simulink model "model_0"  (R2023b)
settings: Solver=VariableStepAuto  StartTime=0.0  StopTime=50  RelTol=1e-3
values from neighbouring files (symbols this model uses):
  is_zero = false    [init.m]
  k_0 = 1    [init.m]    (also in init8.m = 7)
  k_M_0 = 25    [init.m]    (also in init8.m)
  k_M_1 = 10    [init.m]    (also in init8.m)
settings Model: Creator=lalayants  LastModifiedBy=lalayants

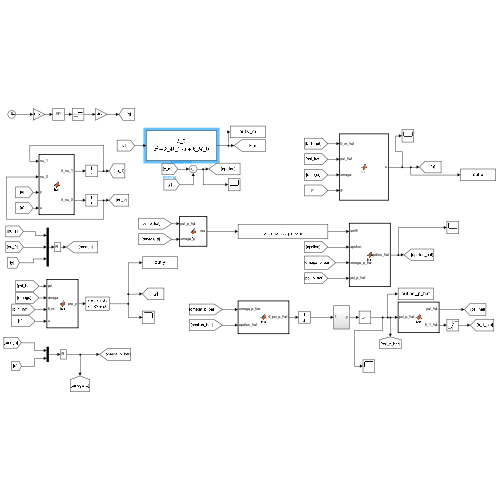
[thumbnail: Simulink's stored preview of the top-level diagram]
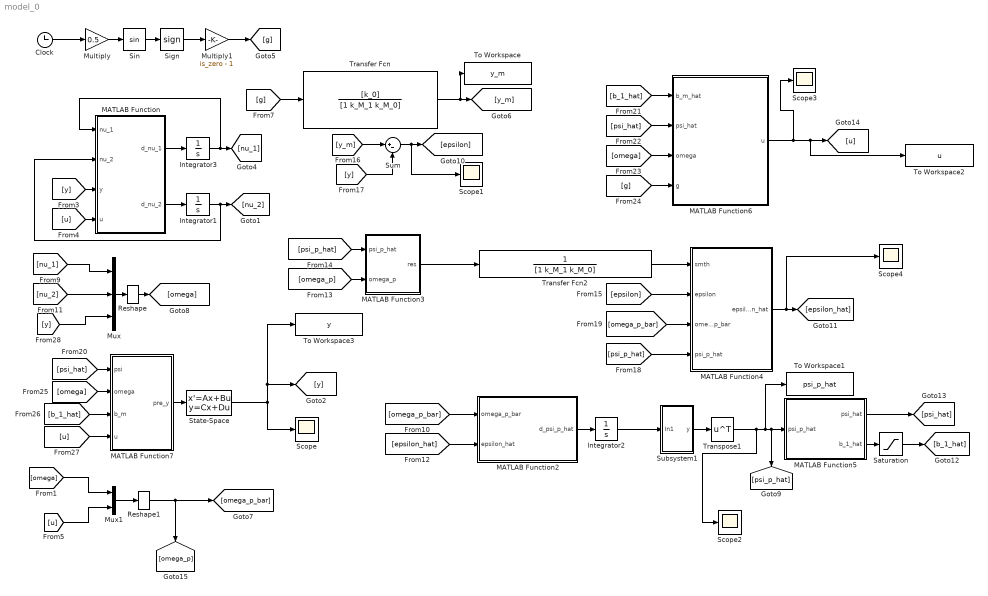
== system model_0 ==
  Clock : Clock
  Integrator1 : Integrator
  Integrator2 : Integrator  InitialCondition=[10; 10; 10; 10]
  Integrator3 : Integrator
  MATLAB Function : MATLAB Function  TreatAsAtomicUnit=on
  MATLAB Function2 : MATLAB Function  TreatAsAtomicUnit=on
  MATLAB Function3 : MATLAB Function  TreatAsAtomicUnit=on
  MATLAB Function4 : MATLAB Function  TreatAsAtomicUnit=on
  MATLAB Function5 : MATLAB Function  TreatAsAtomicUnit=on
  MATLAB Function6 : MATLAB Function  TreatAsAtomicUnit=on
  MATLAB Function7 : MATLAB Function  TreatAsAtomicUnit=on
  Multiply : Gain  Gain=0.5
  Multiply1 : Gain  Gain=is_zero - 1
  Mux : Mux  Inputs=3
  Mux1 : Mux  Inputs=2
  Reshape : Reshape  OutputDimensionality=Customize  OutputDimensions=[3,1]
  Reshape1 : Reshape  OutputDimensionality=Customize  OutputDimensions=[4,1]
  Saturation : Saturate  UpperLimit=1e9  LowerLimit=0.1
  Scope{,1..4} (5 alike) : Scope
  Sign : Signum
  Sin : Trigonometry
  State-Space : StateSpace  A=ss(tf([1], [k_M_1 k_M_0])).A  B=ss(tf([1], [k_M_1 k_M_0])).B  C=ss(tf([1], [k_M_1 k_M_0])).C  D=ss(tf([1], [k_M_1 k_M_0])).D  InitialCondition=1
  Subsystem1 : Subsystem
  Sum : Sum  Inputs=|+-
  To Workspace : ToWorkspace  VariableName=y_m  SaveFormat=Timeseries  SampleTime=-1
  To Workspace1 : ToWorkspace  VariableName=psi_p_hat  SaveFormat=Timeseries  SampleTime=-1
  To Workspace2 : ToWorkspace  VariableName=u  SaveFormat=Timeseries  SampleTime=-1
  To Workspace3 : ToWorkspace  VariableName=y  SaveFormat=Timeseries  SampleTime=-1
  Transfer Fcn : TransferFcn  Numerator=[k_0]  Denominator=[1 k_M_1 k_M_0]
  Transfer Fcn2 : TransferFcn  Denominator=[1 k_M_1 k_M_0]
  Transpose1 : Math  Operator=transpose
  wires:
  [y] -> MATLAB Function/3(y)
  Transfer Fcn/1 -> To Workspace/1, [y_m]
  [g] -> Transfer Fcn/1
  MATLAB Function2/1(d_psi_p_hat) -> Integrator2/1
  Integrator2/1 -> Subsystem1/1(In1)
  [omega_p_bar] -> MATLAB Function2/1(omega_p_bar)
  [epsilon_hat] -> MATLAB Function2/2(epsilon_hat)
  MATLAB Function3/1(res) -> Transfer Fcn2/1
  [y_m] -> Sum/1
  [y] -> Sum/2
  Sum/1 -> Scope1/1, [epsilon]
  [omega_p] -> MATLAB Function3/2(omega_p)
  [psi_p_hat] -> MATLAB Function3/1(psi_p_hat)
  [epsilon] -> MATLAB Function4/2(epsilon)
  Transfer Fcn2/1 -> MATLAB Function4/1(smth)
  [omega_p_bar] -> MATLAB Function4/3(omega_p_bar)
  [psi_p_hat] -> MATLAB Function4/4(psi_p_hat)
  MATLAB Function4/1(epsilon_hat) -> Scope4/1, [epsilon_hat]
  MATLAB Function5/2(b_1_hat) -> Saturation/1
  Saturation/1 -> [b_1_hat]
  MATLAB Function5/1(psi_hat) -> [psi_hat]
  [b_1_hat] -> MATLAB Function6/1(b_m_hat)
  [psi_hat] -> MATLAB Function6/2(psi_hat)
  [omega] -> MATLAB Function6/3(omega)
  [g] -> MATLAB Function6/4(g)
  MATLAB Function6/1(u) -> Scope3/1, To Workspace2/1, [u]
  [psi_hat] -> MATLAB Function7/1(psi)
  [omega] -> MATLAB Function7/2(omega)
  [b_1_hat] -> MATLAB Function7/3(b_m)
  [u] -> MATLAB Function7/4(u)
  Integrator3/1 -> MATLAB Function/1(nu_1), [nu_1]
  [u] -> MATLAB Function/4(u)
  MATLAB Function/1(d_nu_1) -> Integrator3/1
  MATLAB Function/2(d_nu_2) -> Integrator1/1
  [u] -> Mux1/2
  [omega] -> Mux1/1
  Integrator1/1 -> MATLAB Function/2(nu_2), [nu_2]
  [nu_2] -> Mux/2
  [y] -> Mux/3
  Subsystem1/1(y) -> Transpose1/1
  Transpose1/1 -> Scope2/1, To Workspace1/1, MATLAB Function5/1(psi_p_hat), [psi_p_hat]
  Reshape1/1 -> [omega_p_bar], [omega_p]
  Mux/1 -> Reshape/1
  [nu_1] -> Mux/1
  Reshape/1 -> [omega]
  Mux1/1 -> Reshape1/1
  Clock/1 -> Multiply/1
  Sin/1 -> Sign/1
  Sign/1 -> Multiply1/1
  State-Space/1 -> Scope/1, To Workspace3/1, [y]
  MATLAB Function7/1(pre_y) -> State-Space/1
  Multiply/1 -> Sin/1
  Multiply1/1 -> [g]

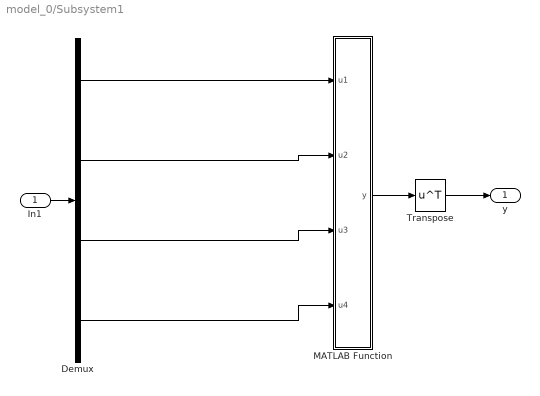
== system model_0/Subsystem1 ==
  In1 : Inport
  Demux : Demux
  MATLAB Function : MATLAB Function  TreatAsAtomicUnit=on
  Transpose : Math  Operator=transpose
  y : Outport
  wires:
  Demux/2 -> MATLAB Function/2(u2)
  In1/1 -> Demux/1
  Demux/4 -> MATLAB Function/4(u4)
  Demux/1 -> MATLAB Function/1(u1)
  Demux/3 -> MATLAB Function/3(u3)
  MATLAB Function/1(y) -> Transpose/1
  Transpose/1 -> y/1

== matlab function model_0/MATLAB Function ==
  data: nu_1 input; nu_2 input; y input; u input; d_nu_1 output; d_nu_2 output; Lambda parameter
function [d_nu_1, d_nu_2]= fcn(nu_1, nu_2, y, u,Lambda)

d_nu_1 = Lambda * nu_1 + u(1);
d_nu_2 = Lambda * nu_2 + y;
% omega = transpose([nu_1 nu_2 y]);
% omega_p = -transpose([transpose(omega) u]);

== matlab function model_0/MATLAB Function2 ==
  data: d_psi_p_hat output; omega_p_bar input; epsilon_hat input; gamma parameter
function d_psi_p_hat = fcn(omega_p_bar, epsilon_hat, gamma)

d_psi_p_hat = gamma * omega_p_bar / (1 + transpose(omega_p_bar) * omega_p_bar) * epsilon_hat;
% d_psi_p_hat = transpose(d_psi_p_hat);

== matlab function model_0/MATLAB Function3 ==
  data: psi_p_hat input; res output; omega_p input
function res = fcn(psi_p_hat, omega_p)

res = transpose(psi_p_hat) * omega_p;

== matlab function model_0/MATLAB Function4 ==
  data: smth input; epsilon_hat output; epsilon input; omega_p_bar input; psi_p_hat input
function epsilon_hat = fcn(smth, epsilon, omega_p_bar, psi_p_hat)

epsilon_hat = epsilon + smth;
epsilon_hat = epsilon + smth - transpose(psi_p_hat) * omega_p_bar;

== matlab function model_0/MATLAB Function5 ==
  data: psi_p_hat input; psi_hat output; b_1_hat output
function [psi_hat, b_1_hat]= fcn(psi_p_hat) 

psi_hat = psi_p_hat(1:3);
b_1_hat = psi_p_hat(4);

== matlab function model_0/MATLAB Function6 ==
  data: b_m_hat input; u output; psi_hat input; omega input; g input; k_0 parameter
function u = fcn(b_m_hat, psi_hat, omega, g, k_0)

u = (-transpose(psi_hat) * omega + k_0 * g) / b_m_hat;

== matlab function model_0/MATLAB Function7 ==
  data: psi input; omega input; b_m input; u input; pre_y output
function pre_y = fcn(psi, omega, b_m, u)

pre_y = transpose(psi) * omega + b_m * u;

== matlab function model_0/Subsystem1/MATLAB Function ==
  data: u1 input; y output; u2 input; u3 input; u4 input
function y = fcn(u1, u2, u3, u4)

y = [u1; u2; u3; u4];
